simulink model "sistemanl_tanques"  (R2018a)
settings: Solver=VariableStepAuto  StartTime=0.0  StopTime=16  RelTol=1e-3
InitFcn:
  | tanques_linealizado
values from neighbouring files (symbols this model uses):
  A = 10    [tanques_lineal_non_lineal.m]
  h1e = 2*h2e    [tanques_lineal_non_lineal.m]
  h2e = (Q/k)^2    [tanques_lineal_non_lineal.m]
undefined symbols (not defined in the file or in its folder): B, C, D, ue
settings Model: Creator=cmparedes  LastModifiedBy=carma

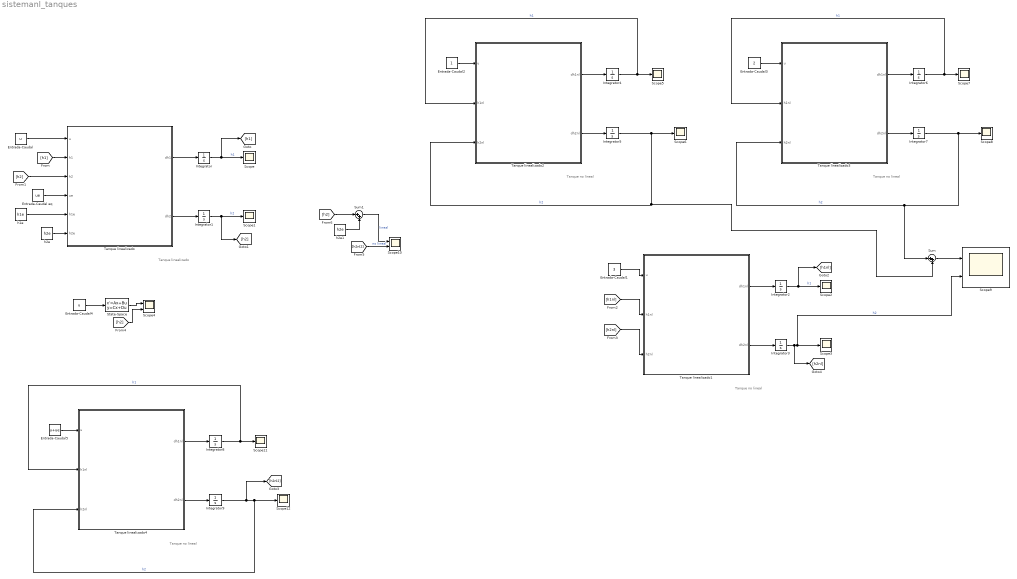
== system sistemanl_tanques ==
  note: Tanque linealizado
  note: Tanque no lineal
  note: Tanque no lineal
  note: Tanque no lineal
  note: Tanque no lineal
  Entrada-Caudal : Constant  Value=u
  Entrada-Caudal eq : Constant  Value=ue
  Entrada-Caudal1 : Constant  Value=3
  Entrada-Caudal2 : Constant
  Entrada-Caudal3 : Constant  Value=2
  Entrada-Caudal4 : Constant  Value=u
  Entrada-Caudal5 : Constant  Value=u+ue
  Integrator : Integrator  InitialCondition=1.1*h1e-h1e
  Integrator1 : Integrator  InitialCondition=1.1*h2e-h2e
  Integrator2 : Integrator  InitialCondition=0.001
  Integrator3 : Integrator
  Integrator4 : Integrator  InitialCondition=0.001  UpperSaturationLimit=2  LowerSaturationLimit=0
  Integrator5 : Integrator
  Integrator6 : Integrator  InitialCondition=0.001  UpperSaturationLimit=2  LowerSaturationLimit=0
  Integrator7 : Integrator
  Integrator8 : Integrator  InitialCondition=1.1*h1e  UpperSaturationLimit=2  LowerSaturationLimit=0
  Integrator9 : Integrator  InitialCondition=1.1*h2e
  Scope{,1..3,5..8,11..12} (10 alike) : Scope
  Scope10 : Scope  NumInputPorts=2
  Scope4 : Scope  NumInputPorts=2
  Scope9 : Scope  NumInputPorts=2
  State-Space : StateSpace  A=A  B=B  C=C  D=D  InitialCondition=[1.1*h1e-h1e;1.1*h2e-h2e]
  Sum : Sum  Inputs=|++
  Sum1 : Sum  Inputs=|++
  Tanque linealizado : MATLAB Function  TreatAsAtomicUnit=on
  Tanque linealizado1 : MATLAB Function  TreatAsAtomicUnit=on
  Tanque linealizado2 : MATLAB Function  TreatAsAtomicUnit=on
  Tanque linealizado3 : MATLAB Function  TreatAsAtomicUnit=on
  Tanque linealizado4 : MATLAB Function  TreatAsAtomicUnit=on
  h1e : Constant  Value=h1e
  h2e : Constant  Value=h2e
  h2e1 : Constant  Value=h2e
  wires:
  Tanque linealizado/1(dh1) -> Integrator/1
  Tanque linealizado/2(dh2) -> Integrator1/1
  Integrator/1 -> [h1], Scope/1  "h1"
  Integrator1/1 -> [h2], Scope1/1  "h2"
  Entrada-Caudal/1 -> Tanque linealizado/1(u)
  [h1] -> Tanque linealizado/2(h1)
  [h2] -> Tanque linealizado/3(h2)
  Entrada-Caudal eq/1 -> Tanque linealizado/4(ue)
  h1e/1 -> Tanque linealizado/5(h1e)
  h2e/1 -> Tanque linealizado/6(h2e)
  Tanque linealizado1/2(dh2nl) -> Integrator3/1
  Tanque linealizado1/1(dh1nl) -> Integrator2/1
  [h1nl] -> Tanque linealizado1/2(h1nl)
  Integrator3/1 -> [h2nl], Scope9/2, Scope3/1  "h2"
  Integrator2/1 -> [h1nl], Scope2/1  "h1"
  Entrada-Caudal1/1 -> Tanque linealizado1/1(u)
  [h2nl] -> Tanque linealizado1/3(h2nl)
  Integrator4/1 -> Tanque linealizado2/2(h1nl), Scope5/1  "h1"
  Integrator5/1 -> Sum/2, Tanque linealizado2/3(h2nl), Scope6/1  "h2"
  Tanque linealizado2/2(dh2nl) -> Integrator5/1
  Entrada-Caudal2/1 -> Tanque linealizado2/1(u)
  Tanque linealizado2/1(dh1nl) -> Integrator4/1
  Tanque linealizado3/1(dh1nl) -> Integrator6/1
  Integrator7/1 -> Sum/1, Tanque linealizado3/3(h2nl), Scope8/1  "h2"
  Integrator6/1 -> Tanque linealizado3/2(h1nl), Scope7/1  "h1"
  Tanque linealizado3/2(dh2nl) -> Integrator7/1
  Entrada-Caudal3/1 -> Tanque linealizado3/1(u)
  Sum/1 -> Scope9/1
  [h2nl2] -> Scope10/2  "no lineal"
  Sum1/1 -> Scope10/1  "lineal"
  [h2] -> Sum1/1
  h2e1/1 -> Sum1/2
  Tanque linealizado4/1(dh1nl) -> Integrator8/1
  Integrator9/1 -> [h2nl2], Tanque linealizado4/3(h2nl), Scope12/1  "h2"
  Tanque linealizado4/2(dh2nl) -> Integrator9/1
  Integrator8/1 -> Tanque linealizado4/2(h1nl), Scope11/1  "h1"
  Entrada-Caudal5/1 -> Tanque linealizado4/1(u)
  Entrada-Caudal4/1 -> State-Space/1
  State-Space/1 -> Scope4/1
  [h2] -> Scope4/2

== matlab function sistemanl_tanques/Tanque linealizado1 ==
  data: u input; dh1nl output; h1nl input; h2nl input; dh2nl output
function [dh1nl,dh2nl] = fcn(u,h1nl,h2nl)


dh1nl=(u-sqrt(h1nl))/(h1nl)^2;
dh2nl=sqrt(h1nl)-sqrt(h2nl);

== matlab function sistemanl_tanques/Tanque linealizado ==
  data: u input; dh1 output; h1 input; h2 input; ue input; h1e input; h2e input; dh2 output
function [dh1,dh2] = fcn(u,h1,h2,ue,h1e,h2e)


%Matriz A jacobiana
A=[(-0.5*h1e^(-0.5)*h1e^2-2*h1e*(ue-sqrt(h1e)))/h1e^4               0;
    0.5*h1e^(-0.5)                                          -0.5*h2e^(-0.5)];
%Matriz B jacobiana
B=[1/h1e^2 ; 0];
h=[h1;h2];

dh=A*h+B*u;

dh1=dh(1,1);
dh2=dh(2,1);

% dh1=h1*(-0.5*h1e^(-0.5)*h1e^2-2*h1e*(ue-sqrt(h1e)))/h1e^4
% dh2= h1*0.5*h1e^(-0.5) -h2*0.5*h2e^(-0.5);

== matlab function sistemanl_tanques/Tanque linealizado2 ==
  data: u input; dh1nl output; h1nl input; h2nl input; dh2nl output
function [dh1nl,dh2nl] = fcn(u,h1nl,h2nl)



dh1nl=(u-sqrt(h1nl))/(h1nl)^2;
dh2nl=sqrt(h1nl)-sqrt(h2nl);

== matlab function sistemanl_tanques/Tanque linealizado3 ==
  data: u input; dh1nl output; h1nl input; h2nl input; dh2nl output
function [dh1nl,dh2nl] = fcn(u,h1nl,h2nl)


dh1nl=(u-sqrt(h1nl))/(h1nl)^2;
dh2nl=sqrt(h1nl)-sqrt(h2nl);

== matlab function sistemanl_tanques/Tanque linealizado4 ==
  data: u input; dh1nl output; h1nl input; h2nl input; dh2nl output
function [dh1nl,dh2nl] = fcn(u,h1nl,h2nl)



dh1nl=(u-sqrt(h1nl))/(h1nl)^2;
dh2nl=sqrt(h1nl)-sqrt(h2nl);
